simulink model "control"  (R2014a)
settings: Solver=ode1  StartTime=0.0  StopTime=inf  FixedStep=Ts  RelTol=1e-3
InitFcn:
  | control_initfcn
StopFcn:
  | control_stopfcn
values from neighbouring files (symbols this model uses):
  armSide = 0    [control_initfcn.m]
  dataLoggerStartTime = 1    [control_initfcn.m]
  dataLoggerStopTime = 100    [control_initfcn.m]
  forgettingFactor = 1e-2    (= 0.01)    [control_initfcn.m]
  g = [0 0 -9.81]'    [control_initfcn.m]
  initializationTime = timeForMovement + 4    (= 9)    [control_initfcn.m]
  initOrientationLeftArmTwo = [1 0 0 0]    [control_initfcn.m]
  initOrientationRightArmTwo = [1 0 0 0]    [control_initfcn.m]
  initPositionLeftArm = [0.7 0.23 1]    [control_initfcn.m]
  initPositionRightArm = [0.7 -0.23 1]    [control_initfcn.m]
  MANIPULATION_CMD_CONFIGURATION = 6    [control_initfcn.m]
  MANIPULATION_CMD_CONFIGURATION_VELOCITY = 102    [control_initfcn.m]
  maxTime = 10    [control_initfcn.m]
  minTime = 0.1    [control_initfcn.m]
  rampTime = 2    [control_initfcn.m]
  rotationAmplitude = [0.15;0;0.1462]    [control_initfcn.m]
  rotationFrequency = [0.5;0.6283;1.0472]    [control_initfcn.m]
  rotationPhaseShift = [pi;0;0]    [control_initfcn.m]
  timeForMovement = 5    [control_initfcn.m]
  translationAmplitude = 0*[0.005;0.02;0.01]    [control_initfcn.m]
  translationFrequency = [1.0472;0.6283;1.0472]    [control_initfcn.m]
  translationPhaseShift = [pi;0;0]    [control_initfcn.m]
  Ts = 0.01    [control_initfcn.m]
  vxMax = 0.5    [control_initfcn.m]
  vyMax = 0.5    [control_initfcn.m]
  vzMax = 0.5    [control_initfcn.m]
  wxMax = 0.5    [control_initfcn.m]
  wyMax = 0.5    [control_initfcn.m]
  wzMax = 0.5    [control_initfcn.m]
  xMax = 0.5 + offsetx    (= 1.2)    [control_initfcn.m]
  xMin = -0.1 + offsetx    (= 0.6)    [control_initfcn.m]
  yMax = 0.5 + offsety    (= 0.27)    [control_initfcn.m]
  yMin = -0.5 + offsety    (= -0.73)    [control_initfcn.m]
  zMax = 0.5 + offsetz    (= 1.4)    [control_initfcn.m]
  zMin = -0.5 + offsetz    (= 0.4)    [control_initfcn.m]
undefined symbols (not defined in the file or in its folder): cobot1a, qualisys, ws
libraries: dsparch4 x27, rtai_devices x22, sfbc_lib x6, simulink x2, rtai_utilities x2
settings Model: SimulationMode=external  Creator=wirnshofer  LastModifiedBy=bschmidt
settings DataIOCC: SignalLoggingSaveFormat=ModelDataLogs
settings RTWCC: SystemTargetFile=prt.tlc  TemplateMakefile=prt.tmf  Description=Linux PREEMPT_RT Real-Time Target  ProcessScript=prt_make_rtw_hook
settings STFCustomTargetCC: TargetLangStandard=C99 (ISO)  CodeReplacementLibrary=GNU C99 extensions  ModelReferenceCompliant=off  ConcurrentExecutionCompliant=off  MatFileLogging=on  SystemTargetFile=prt.tlc
settings GRTTargetCC: TargetLangStandard=C99 (ISO)  CodeReplacementLibrary=GNU C99 extensions  ModelReferenceCompliant=off  ParMdlRefBuildCompliant=off  CompOptLevelCompliant=off  ConcurrentExecutionCompliant=off  CombineOutputUpdateFcns=off  CPPClassGenCompliant=off  GRTInterface=on  ExtMode=on  ExtModeMexArgs='cobot1b'

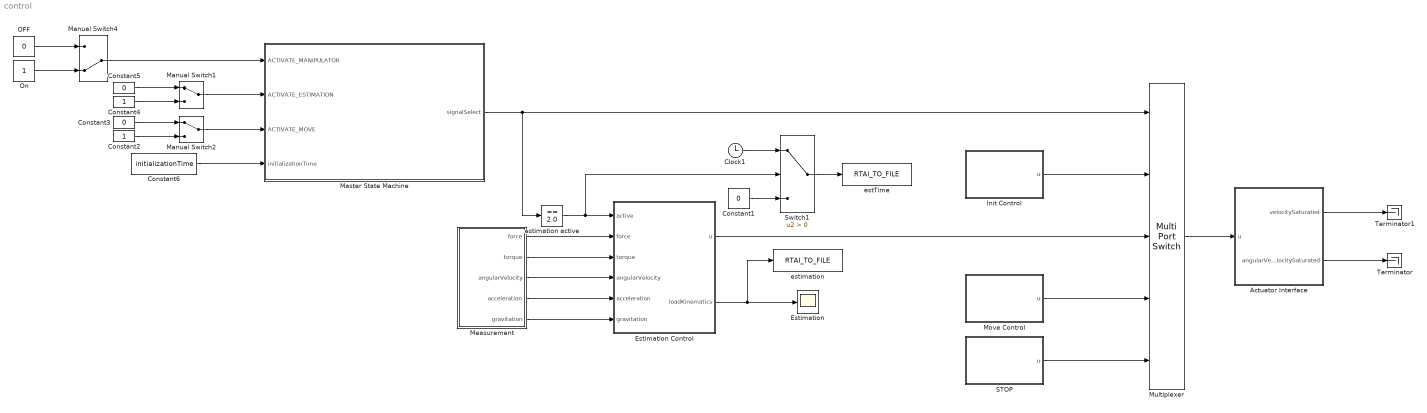
== system control ==
  Actuator Interface : Subsystem
  Clock1 : Clock
  Constant1 : Constant  Value=0
  Constant2 : Constant
  Constant3 : Constant  Value=0
  Constant4 : Constant
  Constant5 : Constant  Value=0
  Constant6 : Constant  Value=initializationTime
  Estimation : Scope
  Estimation Control : Subsystem
  Init Control : Subsystem
  Manual Switch1 : ManualSwitch
  Manual Switch2 : ManualSwitch
  Manual Switch4 : ManualSwitch  CurrentSetting=0
  Master State Machine : Stateflow chart  TreatAsAtomicUnit=on
  Measurement : Subsystem
  Move Control : Subsystem
  Multiplexer : MultiPortSwitch  Inputs=4
  OFF : Constant  Value=0
  On : Constant
  STOP : Subsystem
  Switch1 : Switch  Criteria=u2 > Threshold
  Terminator : Terminator
  Terminator1 : Terminator
  estTime : rtai_devices/RTAI_TO_FILE  N=1  InType=double  FileName='estTime.dat'  FpOutStr='%f '  TStartStop=[dataLoggerStartTime dataLoggerStopTime]  T=Ts  Confirm=off  Cutoff=off
  estimation : rtai_devices/RTAI_TO_FILE  N=10  InType=double  FileName='estimation.dat'  FpOutStr='%f '  TStartStop=[dataLoggerStartTime dataLoggerStopTime]  T=Ts  Confirm=off  Cutoff=off
  estimation active : simulink/Logic and Bit Operations/Compare To Constant  relop===  const=2.0  OutDataTypeStr=boolean
  wires:
  Init Control/1(u) -> Multiplexer/2
  Estimation Control/1(u) -> Multiplexer/3
  STOP/1(u) -> Multiplexer/5
  Move Control/1(u) -> Multiplexer/4
  Multiplexer/1 -> Actuator Interface/1(u)
  OFF/1 -> Manual Switch4/1
  On/1 -> Manual Switch4/2
  Manual Switch2/1 -> Master State Machine/3(ACTIVATE_MOVE)
  Constant3/1 -> Manual Switch2/1
  Constant2/1 -> Manual Switch2/2
  Estimation Control/2(loadKinematics) -> estimation/1, Estimation/1
  Measurement/1(force) -> Estimation Control/2(force)
  Measurement/2(torque) -> Estimation Control/3(torque)
  Measurement/5(gravitation) -> Estimation Control/6(gravitation)
  Measurement/3(angularVelocity) -> Estimation Control/4(angularVelocity)
  Actuator Interface/2(angularVelocitySaturated) -> Terminator/1
  Actuator Interface/1(velocitySaturated) -> Terminator1/1
  Measurement/4(acceleration) -> Estimation Control/5(acceleration)
  Manual Switch4/1 -> Master State Machine/1(ACTIVATE_MANIPULATOR)
  Switch1/1 -> estTime/1
  Manual Switch1/1 -> Master State Machine/2(ACTIVATE_ESTIMATION)
  Constant5/1 -> Manual Switch1/1
  Constant4/1 -> Manual Switch1/2
  Master State Machine/1(signalSelect) -> Multiplexer/1, estimation active/1
  estimation active/1 -> Switch1/2, Estimation Control/1(active)
  Constant1/1 -> Switch1/3
  Clock1/1 -> Switch1/1
  Constant6/1 -> Master State Machine/4(initializationTime)

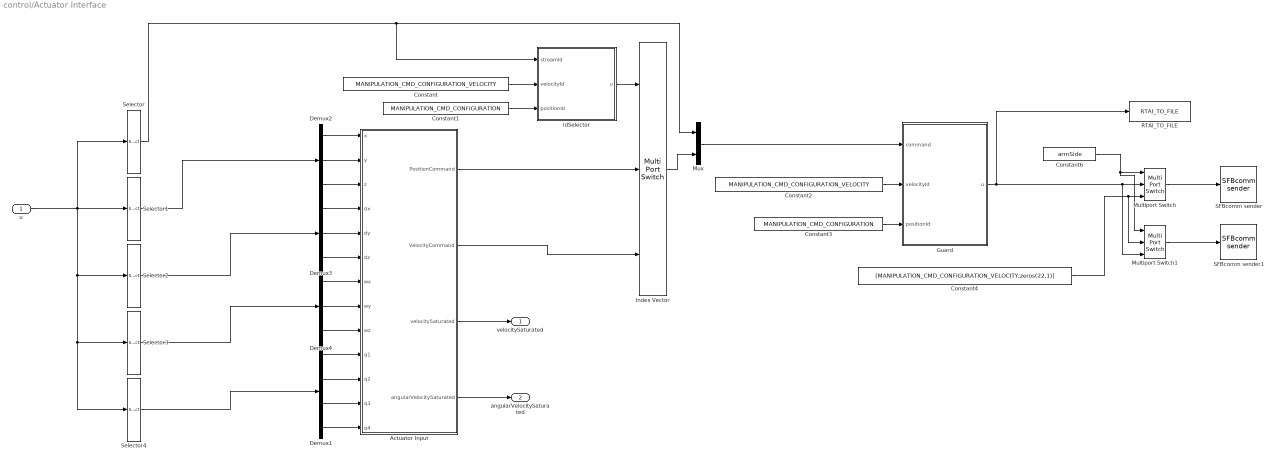
== system control/Actuator Interface ==
  u : Inport
  Actuator Input : Subsystem
  Constant : Constant  Value=MANIPULATION_CMD_CONFIGURATION_VELOCITY
  Constant1 : Constant  Value=MANIPULATION_CMD_CONFIGURATION
  Constant2 : Constant  Value=MANIPULATION_CMD_CONFIGURATION_VELOCITY
  Constant3 : Constant  Value=MANIPULATION_CMD_CONFIGURATION
  Constant4 : Constant  Value=[MANIPULATION_CMD_CONFIGURATION_VELOCITY;zeros(22,1)]
  Constant6 : Constant  Value=armSide
  Demux1 : Demux
  Demux2 : Demux  Outputs=3
  Demux3 : Demux  Outputs=3
  Demux4 : Demux  Outputs=3
  Guard : MATLAB Function  TreatAsAtomicUnit=on
  IdSelector : MATLAB Function  TreatAsAtomicUnit=on
  Index Vector : MultiPortSwitch  DataPortOrder=Zero-based contiguous  Inputs=2  zeroidx=on
  Multiport Switch : MultiPortSwitch  DataPortOrder=Zero-based contiguous  Inputs=2
  Multiport Switch1 : MultiPortSwitch  DataPortOrder=Zero-based contiguous  Inputs=2
  Mux : Mux  Inputs=2
  RTAI_TO_FILE : rtai_devices/RTAI_TO_FILE  N=23  InType=double  FileName='actContCmd.dat'  FpOutStr='%f '  TStartStop=[dataLoggerStartTime dataLoggerStopTime]  T=Ts  Confirm=off  Cutoff=off
  SFBcomm sender : sfbc_lib/SFBcomm sender  localPort=8566  streamID=2  remoteSettings=cobot1a:8565  portNames=A  connectTimeout=200  sampleTime=-1
  SFBcomm sender1 : sfbc_lib/SFBcomm sender  localPort=7566  streamID=2  remoteSettings=cobot1a:7565  portNames=A  connectTimeout=200  sampleTime=-1
  Selector : Selector  InputPortWidth=14
  Selector1 : Selector  InputPortWidth=14  Indices=[2:4]
  Selector2 : Selector  InputPortWidth=14  Indices=[5:7]
  Selector3 : Selector  InputPortWidth=14  Indices=[8:10]
  Selector4 : Selector  InputPortWidth=14  Indices=[11:14]
  velocitySaturated : Outport
  angularVelocitySaturated : Outport  Port=2
  wires:
  Constant/1 -> IdSelector/2(velocityId)
  Actuator Input/1(PositionCommand) -> Index Vector/2
  Constant1/1 -> IdSelector/3(positionId)
  Constant3/1 -> Guard/3(positionId)
  IdSelector/1(u) -> Index Vector/1
  Selector/1 -> IdSelector/1(streamId), Mux/1
  Mux/1 -> Guard/1(command)
  Index Vector/1 -> Mux/2
  Actuator Input/2(VelocityCommand) -> Index Vector/3
  Constant2/1 -> Guard/2(velocityId)
  u/1 -> Selector/1, Selector4/1, Selector3/1, Selector2/1, Selector1/1
  Demux2/3 -> Actuator Input/3(z)
  Demux2/1 -> Actuator Input/1(x)
  Demux2/2 -> Actuator Input/2(y)
  Demux3/1 -> Actuator Input/4(dx)
  Demux3/2 -> Actuator Input/5(dy)
  Demux3/3 -> Actuator Input/6(dz)
  Demux4/2 -> Actuator Input/8(wy)
  Demux4/1 -> Actuator Input/7(wx)
  Demux4/3 -> Actuator Input/9(wz)
  Selector1/1 -> Demux2/1
  Selector2/1 -> Demux3/1
  Selector3/1 -> Demux4/1
  Demux1/1 -> Actuator Input/10(q1)
  Demux1/2 -> Actuator Input/11(q2)
  Demux1/3 -> Actuator Input/12(q3)
  Demux1/4 -> Actuator Input/13(q4)
  Selector4/1 -> Demux1/1
  Actuator Input/3(velocitySaturated) -> velocitySaturated/1
  Actuator Input/4(angularVelocitySaturated) -> angularVelocitySaturated/1
  Multiport Switch1/1 -> SFBcomm sender1/1
  Guard/1(u) -> Multiport Switch1/3, Multiport Switch/2, RTAI_TO_FILE/1
  Multiport Switch/1 -> SFBcomm sender/1
  Constant4/1 -> Multiport Switch1/2, Multiport Switch/3
  Constant6/1 -> Multiport Switch1/1, Multiport Switch/1

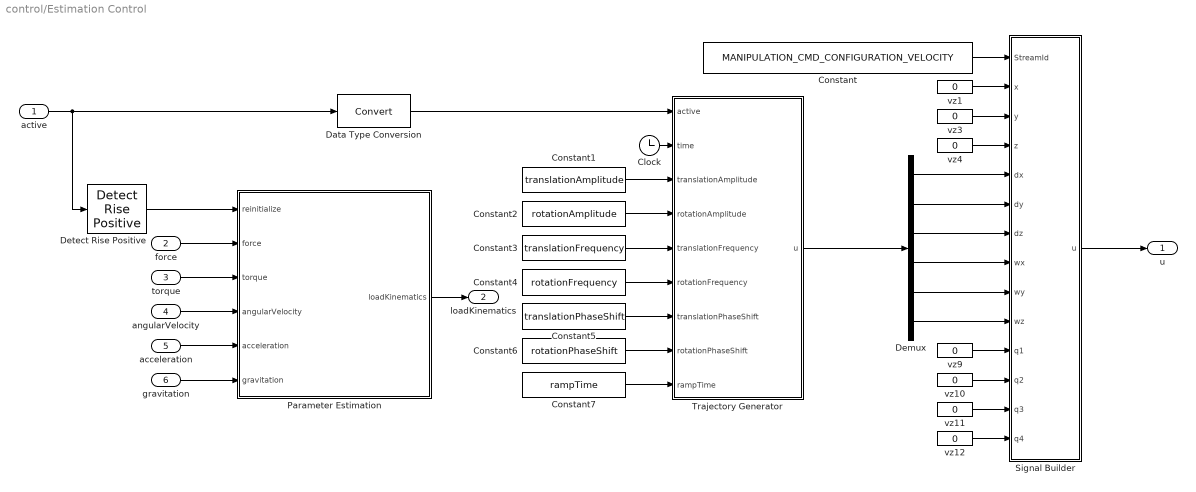
== system control/Estimation Control ==
  active : Inport
  force : Inport  Port=2
  torque : Inport  Port=3
  angularVelocity : Inport  Port=4
  acceleration : Inport  Port=5
  gravitation : Inport  Port=6
  Clock : Clock
  Constant : Constant  Value=MANIPULATION_CMD_CONFIGURATION_VELOCITY
  Constant1 : Constant  Value=translationAmplitude
  Constant2 : Constant  Value=rotationAmplitude
  Constant3 : Constant  Value=translationFrequency
  Constant4 : Constant  Value=rotationFrequency
  Constant5 : Constant  Value=translationPhaseShift
  Constant6 : Constant  Value=rotationPhaseShift
  Constant7 : Constant  Value=rampTime
  Data Type Conversion : DataTypeConversion
  Demux : Demux  Outputs=6
  Detect Rise Positive : simulink/Logic and Bit Operations/Detect Rise Positive  vinit=0  InputProcessing=Inherited  OutDataTypeStr=boolean
  Parameter Estimation : Subsystem
  Signal Builder : Subsystem
  Trajectory Generator : MATLAB Function  TreatAsAtomicUnit=on
  vz{1,3..4,9..12} (7 alike) : Constant  Value=0  SampleTime=Ts
  u : Outport
  loadKinematics : Outport  Port=2
  wires:
  active/1 -> Data Type Conversion/1, Detect Rise Positive/1
  Detect Rise Positive/1 -> Parameter Estimation/1(reinitialize)
  Constant/1 -> Signal Builder/1(StreamId)
  vz1/1 -> Signal Builder/2(x)
  vz3/1 -> Signal Builder/3(y)
  vz9/1 -> Signal Builder/11(q1)
  vz10/1 -> Signal Builder/12(q2)
  vz11/1 -> Signal Builder/13(q3)
  vz12/1 -> Signal Builder/14(q4)
  Signal Builder/1(u) -> u/1
  acceleration/1 -> Parameter Estimation/5(acceleration)
  angularVelocity/1 -> Parameter Estimation/4(angularVelocity)
  force/1 -> Parameter Estimation/2(force)
  torque/1 -> Parameter Estimation/3(torque)
  gravitation/1 -> Parameter Estimation/6(gravitation)
  Parameter Estimation/1(loadKinematics) -> loadKinematics/1
  vz4/1 -> Signal Builder/4(z)
  Clock/1 -> Trajectory Generator/2(time)
  Constant1/1 -> Trajectory Generator/3(translationAmplitude)
  Constant2/1 -> Trajectory Generator/4(rotationAmplitude)
  Constant6/1 -> Trajectory Generator/8(rotationPhaseShift)
  Constant3/1 -> Trajectory Generator/5(translationFrequency)
  Constant4/1 -> Trajectory Generator/6(rotationFrequency)
  Constant5/1 -> Trajectory Generator/7(translationPhaseShift)
  Constant7/1 -> Trajectory Generator/9(rampTime)
  Demux/6 -> Signal Builder/10(wz)
  Demux/5 -> Signal Builder/9(wy)
  Demux/4 -> Signal Builder/8(wx)
  Demux/3 -> Signal Builder/7(dz)
  Demux/2 -> Signal Builder/6(dy)
  Demux/1 -> Signal Builder/5(dx)
  Trajectory Generator/1(u) -> Demux/1
  Data Type Conversion/1 -> Trajectory Generator/1(active)

== system control/Init Control ==
  Constant : Constant  Value=armSide
  Constant1 : Constant  Value=initOrientationRightArmTwo
  Constant2 : Constant  Value=MANIPULATION_CMD_CONFIGURATION
  Constant3 : Constant  Value=zeros(6,1)
  Constant5 : Constant  Value=initPositionRightArm
  Constant6 : Constant  Value=initPositionLeftArm
  Constant7 : Constant  Value=initOrientationLeftArmTwo
  Demux : Demux  Outputs=3
  Demux1 : Demux  Outputs=6
  Demux2 : Demux
  Multiport Switch : MultiPortSwitch  DataPortOrder=Zero-based contiguous  Inputs=2
  Multiport Switch1 : MultiPortSwitch  DataPortOrder=Zero-based contiguous  Inputs=2
  Signal Builder : Subsystem
  u : Outport
  wires:
  Signal Builder/1(u) -> u/1
  Constant2/1 -> Signal Builder/1(StreamId)
  Demux/2 -> Signal Builder/3(y)
  Demux/1 -> Signal Builder/2(x)
  Demux/3 -> Signal Builder/4(z)
  Constant5/1 -> Multiport Switch/2
  Constant3/1 -> Demux1/1
  Constant1/1 -> Multiport Switch1/2
  Demux1/1 -> Signal Builder/5(dx)
  Demux1/2 -> Signal Builder/6(dy)
  Demux1/3 -> Signal Builder/7(dz)
  Demux1/4 -> Signal Builder/8(wx)
  Demux1/5 -> Signal Builder/9(wy)
  Demux1/6 -> Signal Builder/10(wz)
  Demux2/1 -> Signal Builder/11(q1)
  Demux2/2 -> Signal Builder/12(q2)
  Demux2/3 -> Signal Builder/13(q3)
  Demux2/4 -> Signal Builder/14(q4)
  Multiport Switch1/1 -> Demux2/1
  Multiport Switch/1 -> Demux/1
  Constant6/1 -> Multiport Switch/3
  Constant7/1 -> Multiport Switch1/3
  Constant/1 -> Multiport Switch1/1, Multiport Switch/1

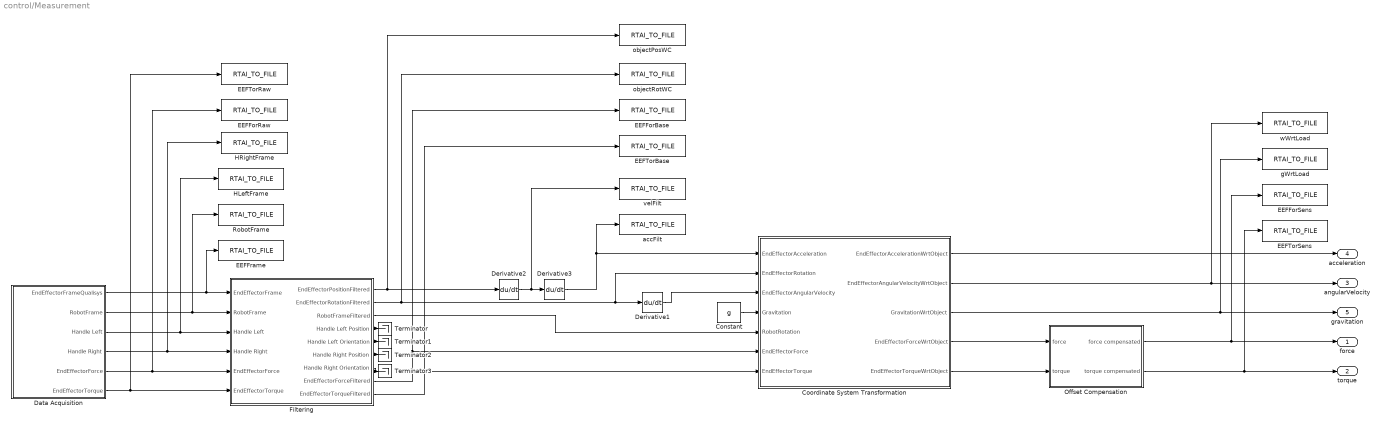
== system control/Measurement ==
  Constant : Constant  Value=g  SampleTime=-1
  Coordinate System Transformation : Subsystem
  Data Acquisition : Subsystem
  Derivative1 : Derivative
  Derivative2 : Derivative
  Derivative3 : Derivative
  EEFForBase : rtai_devices/RTAI_TO_FILE  N=3  InType=double  FileName='EEFForBase.dat'  FpOutStr='%f '  TStartStop=[dataLoggerStartTime dataLoggerStopTime]  T=Ts  Confirm=off  Cutoff=off
  EEFForRaw : rtai_devices/RTAI_TO_FILE  N=3  InType=double  FileName='EEFForRaw.dat'  FpOutStr='%f '  TStartStop=[dataLoggerStartTime dataLoggerStopTime]  T=Ts  Confirm=off  Cutoff=off
  EEFForSens : rtai_devices/RTAI_TO_FILE  N=3  InType=double  FileName='EEFForSens.dat'  FpOutStr='%f '  TStartStop=[dataLoggerStartTime dataLoggerStopTime]  T=Ts  Confirm=off  Cutoff=off
  EEFFrame : rtai_devices/RTAI_TO_FILE  N=8  InType=double  FileName='EEFFrame.dat'  FpOutStr='%f '  TStartStop=[dataLoggerStartTime dataLoggerStopTime]  T=Ts  Confirm=off  Cutoff=off
  EEFTorBase : rtai_devices/RTAI_TO_FILE  N=3  InType=double  FileName='EEFTorBase.dat'  FpOutStr='%f '  TStartStop=[dataLoggerStartTime dataLoggerStopTime]  T=Ts  Confirm=off  Cutoff=off
  EEFTorRaw : rtai_devices/RTAI_TO_FILE  N=3  InType=double  FileName='EEFTorRaw.dat'  FpOutStr='%f '  TStartStop=[dataLoggerStartTime dataLoggerStopTime]  T=Ts  Confirm=off  Cutoff=off
  EEFTorSens : rtai_devices/RTAI_TO_FILE  N=3  InType=double  FileName='EEFTorSens.dat'  FpOutStr='%f '  TStartStop=[dataLoggerStartTime dataLoggerStopTime]  T=Ts  Confirm=off  Cutoff=off
  Filtering : Subsystem
  HLeftFrame : rtai_devices/RTAI_TO_FILE  N=8  InType=double  FileName='HLeftFrame.dat'  FpOutStr='%f '  TStartStop=[dataLoggerStartTime dataLoggerStopTime]  T=Ts  Confirm=off  Cutoff=off
  HRightFrame : rtai_devices/RTAI_TO_FILE  N=8  InType=double  FileName='HRightFrame.dat'  FpOutStr='%f '  TStartStop=[dataLoggerStartTime dataLoggerStopTime]  T=Ts  Confirm=off  Cutoff=off
  Offset Compensation : Subsystem
  RobotFrame : rtai_devices/RTAI_TO_FILE  N=8  InType=double  FileName='RobotFrame.dat'  FpOutStr='%f '  TStartStop=[dataLoggerStartTime dataLoggerStopTime]  T=Ts  Confirm=off  Cutoff=off
  Terminator{,1..3} (4 alike) : Terminator
  accFilt : rtai_devices/RTAI_TO_FILE  N=3  InType=double  FileName='accFilt.dat'  FpOutStr='%f '  TStartStop=[dataLoggerStartTime dataLoggerStopTime]  T=Ts  Confirm=off  Cutoff=off
  gWrtLoad : rtai_devices/RTAI_TO_FILE  N=3  InType=double  FileName='gWrtLoad.dat'  FpOutStr='%f '  TStartStop=[dataLoggerStartTime dataLoggerStopTime]  T=Ts  Confirm=off  Cutoff=off
  objectPosWC : rtai_devices/RTAI_TO_FILE  N=3  InType=double  FileName='objectPosWC.dat'  FpOutStr='%f '  TStartStop=[dataLoggerStartTime dataLoggerStopTime]  T=Ts  Confirm=off  Cutoff=off
  objectRotWC : rtai_devices/RTAI_TO_FILE  N=3  InType=double  FileName='objectRotWC.dat'  FpOutStr='%f '  TStartStop=[dataLoggerStartTime dataLoggerStopTime]  T=Ts  Confirm=off  Cutoff=off
  velFilt : rtai_devices/RTAI_TO_FILE  N=3  InType=double  FileName='velFilt.dat'  FpOutStr='%f '  TStartStop=[dataLoggerStartTime dataLoggerStopTime]  T=Ts  Confirm=off  Cutoff=off
  wWrtLoad : rtai_devices/RTAI_TO_FILE  N=3  InType=double  FileName='wWrtLoad.dat'  FpOutStr='%f '  TStartStop=[dataLoggerStartTime dataLoggerStopTime]  T=Ts  Confirm=off  Cutoff=off
  force : Outport
  torque : Outport  Port=2
  angularVelocity : Outport  Port=3
  acceleration : Outport  Port=4
  gravitation : Outport  Port=5
  wires:
  Derivative2/1 -> Derivative3/1, velFilt/1
  Derivative3/1 -> Coordinate System Transformation/1(EndEffectorAcceleration), accFilt/1
  Filtering/9(EndEffectorTorqueFiltered) -> EEFTorBase/1, Coordinate System Transformation/7(EndEffectorTorque)
  Filtering/8(EndEffectorForceFiltered) -> EEFForBase/1, Coordinate System Transformation/6(EndEffectorForce)
  Filtering/1(EndEffectorPositionFiltered) -> Derivative2/1, objectPosWC/1
  Data Acquisition/1(EndEffectorFrameQualisys) -> EEFFrame/1, Filtering/1(EndEffectorFrame)
  Data Acquisition/2(RobotFrame) -> RobotFrame/1, Filtering/2(RobotFrame)
  Data Acquisition/5(EndEffectorForce) -> EEFForRaw/1, Filtering/5(EndEffectorForce)
  Data Acquisition/6(EndEffectorTorque) -> EEFTorRaw/1, Filtering/6(EndEffectorTorque)
  Coordinate System Transformation/2(EndEffectorAngularVelocityWrtObject) -> angularVelocity/1, wWrtLoad/1
  Coordinate System Transformation/3(GravitationWrtObject) -> gravitation/1, gWrtLoad/1
  Derivative1/1 -> Coordinate System Transformation/3(EndEffectorAngularVelocity)
  Constant/1 -> Coordinate System Transformation/4(Gravitation)
  Filtering/3(RobotFrameFiltered) -> Coordinate System Transformation/5(RobotRotation)
  Coordinate System Transformation/1(EndEffectorAccelerationWrtObject) -> acceleration/1
  Filtering/2(EndEffectorRotationFiltered) -> Derivative1/1, Coordinate System Transformation/2(EndEffectorRotation), objectRotWC/1
  Data Acquisition/3(Handle Left) -> HLeftFrame/1, Filtering/3(Handle Left)
  Data Acquisition/4(Handle Right) -> HRightFrame/1, Filtering/4(Handle Right)
  Filtering/4(Handle Left Position) -> Terminator/1
  Filtering/5(Handle Left Orientation) -> Terminator1/1
  Filtering/6(Handle Right Position) -> Terminator2/1
  Filtering/7(Handle Right Orientation) -> Terminator3/1
  Offset Compensation/2(torque compensated) -> EEFTorSens/1, torque/1
  Offset Compensation/1(force compensated) -> EEFForSens/1, force/1
  Coordinate System Transformation/4(EndEffectorForceWrtObject) -> Offset Compensation/1(force)
  Coordinate System Transformation/5(EndEffectorTorqueWrtObject) -> Offset Compensation/2(torque)

== system control/Move Control ==
  Constant : Constant  Value=MANIPULATION_CMD_CONFIGURATION_VELOCITY
  Signal Builder : Subsystem
  vz{,1..12} (13 alike) : Constant  Value=0  SampleTime=Ts
  u : Outport
  wires:
  vz/1 -> Signal Builder/2(x)
  vz2/1 -> Signal Builder/4(z)
  vz1/1 -> Signal Builder/3(y)
  Constant/1 -> Signal Builder/1(StreamId)
  Signal Builder/1(u) -> u/1
  vz3/1 -> Signal Builder/5(dx)
  vz8/1 -> Signal Builder/10(wz)
  vz5/1 -> Signal Builder/7(dz)
  vz4/1 -> Signal Builder/6(dy)
  vz7/1 -> Signal Builder/9(wy)
  vz6/1 -> Signal Builder/8(wx)
  vz12/1 -> Signal Builder/14(q4)
  vz9/1 -> Signal Builder/11(q1)
  vz11/1 -> Signal Builder/13(q3)
  vz10/1 -> Signal Builder/12(q2)

== system control/STOP ==
  Constant : Constant  Value=MANIPULATION_CMD_CONFIGURATION_VELOCITY
  Constant1 : Constant  Value=zeros(13,1)
  Demux : Demux  Outputs=13
  Signal Builder : Subsystem
  u : Outport
  wires:
  Signal Builder/1(u) -> u/1
  Constant/1 -> Signal Builder/1(StreamId)
  Demux/3 -> Signal Builder/4(z)
  Demux/6 -> Signal Builder/7(dz)
  Demux/1 -> Signal Builder/2(x)
  Demux/5 -> Signal Builder/6(dy)
  Demux/2 -> Signal Builder/3(y)
  Demux/7 -> Signal Builder/8(wx)
  Demux/9 -> Signal Builder/10(wz)
  Demux/8 -> Signal Builder/9(wy)
  Demux/4 -> Signal Builder/5(dx)
  Constant1/1 -> Demux/1
  Demux/10 -> Signal Builder/11(q1)
  Demux/11 -> Signal Builder/12(q2)
  Demux/12 -> Signal Builder/13(q3)
  Demux/13 -> Signal Builder/14(q4)

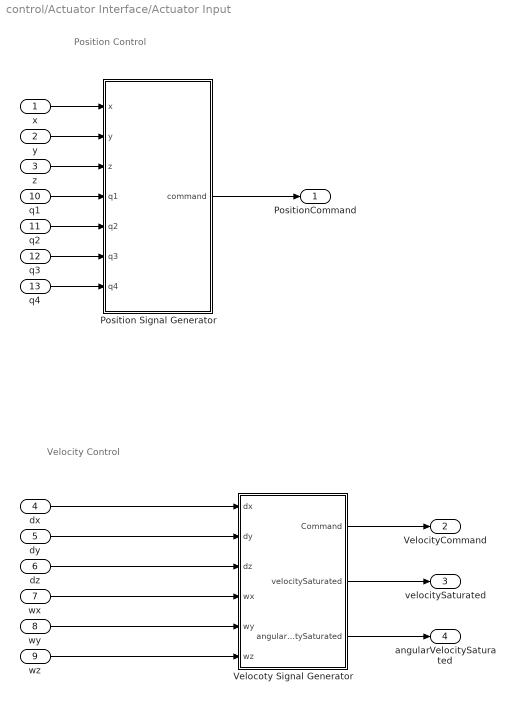
== system control/Actuator Interface/Actuator Input ==
  note: Velocity Control
  note: Position Control
  x : Inport
  y : Inport  Port=2
  z : Inport  Port=3
  dx : Inport  Port=4
  dy : Inport  Port=5
  dz : Inport  Port=6
  wx : Inport  Port=7
  wy : Inport  Port=8
  wz : Inport  Port=9
  q1 : Inport  Port=10
  q2 : Inport  Port=11
  q3 : Inport  Port=12
  q4 : Inport  Port=13
  Position Signal Generator : Subsystem
  Velocoty Signal Generator : Subsystem
  PositionCommand : Outport
  VelocityCommand : Outport  Port=2
  velocitySaturated : Outport  Port=3
  angularVelocitySaturated : Outport  Port=4
  wires:
  y/1 -> Position Signal Generator/2(y)
  Velocoty Signal Generator/1(Command) -> VelocityCommand/1
  wz/1 -> Velocoty Signal Generator/6(wz)
  z/1 -> Position Signal Generator/3(z)
  dx/1 -> Velocoty Signal Generator/1(dx)
  wx/1 -> Velocoty Signal Generator/4(wx)
  Position Signal Generator/1(command) -> PositionCommand/1
  wy/1 -> Velocoty Signal Generator/5(wy)
  dz/1 -> Velocoty Signal Generator/3(dz)
  dy/1 -> Velocoty Signal Generator/2(dy)
  x/1 -> Position Signal Generator/1(x)
  q1/1 -> Position Signal Generator/4(q1)
  q2/1 -> Position Signal Generator/5(q2)
  q3/1 -> Position Signal Generator/6(q3)
  q4/1 -> Position Signal Generator/7(q4)
  Velocoty Signal Generator/2(velocitySaturated) -> velocitySaturated/1
  Velocoty Signal Generator/3(angularVelocitySaturated) -> angularVelocitySaturated/1

== system control/Estimation Control/Parameter Estimation ==
  reinitialize : Inport
  force : Inport  Port=2
  torque : Inport  Port=3
  angularVelocity : Inport  Port=4
  acceleration : Inport  Port=5
  gravitation : Inport  Port=6
  Constant : Constant  Value=forgettingFactor
  Load Dynamics Estimation : MATLAB Function  TreatAsAtomicUnit=on
  anuglarAcceleration : Derivative
  loadKinematics : Outport
  wires:
  angularVelocity/1 -> Load Dynamics Estimation/3(omega), anuglarAcceleration/1
  acceleration/1 -> Load Dynamics Estimation/5(ddp)
  anuglarAcceleration/1 -> Load Dynamics Estimation/4(domega)
  Load Dynamics Estimation/1(thetaHat) -> loadKinematics/1
  force/1 -> Load Dynamics Estimation/1(F)
  torque/1 -> Load Dynamics Estimation/2(N)
  gravitation/1 -> Load Dynamics Estimation/6(g)
  Constant/1 -> Load Dynamics Estimation/7(forgettingFactor)
  reinitialize/1 -> Load Dynamics Estimation/8(reinitialize)

== system control/Estimation Control/Signal Builder ==
  StreamId : Inport
  x : Inport  Port=2
  y : Inport  Port=3
  z : Inport  Port=4
  dx : Inport  Port=5
  dy : Inport  Port=6
  dz : Inport  Port=7
  wx : Inport  Port=8
  wy : Inport  Port=9
  wz : Inport  Port=10
  q1 : Inport  Port=11
  q2 : Inport  Port=12
  q3 : Inport  Port=13
  q4 : Inport  Port=14
  Mux : Mux  Inputs=14
  u : Outport
  wires:
  Mux/1 -> u/1
  wy/1 -> Mux/9
  wx/1 -> Mux/8
  StreamId/1 -> Mux/1
  x/1 -> Mux/2
  dy/1 -> Mux/6
  dz/1 -> Mux/7
  dx/1 -> Mux/5
  z/1 -> Mux/4
  y/1 -> Mux/3
  wz/1 -> Mux/10
  q2/1 -> Mux/12
  q1/1 -> Mux/11
  q3/1 -> Mux/13
  q4/1 -> Mux/14

== system control/Init Control/Signal Builder ==
  StreamId : Inport
  x : Inport  Port=2
  y : Inport  Port=3
  z : Inport  Port=4
  dx : Inport  Port=5
  dy : Inport  Port=6
  dz : Inport  Port=7
  wx : Inport  Port=8
  wy : Inport  Port=9
  wz : Inport  Port=10
  q1 : Inport  Port=11
  q2 : Inport  Port=12
  q3 : Inport  Port=13
  q4 : Inport  Port=14
  Mux : Mux  Inputs=14
  u : Outport
  wires:
  Mux/1 -> u/1
  wy/1 -> Mux/9
  wx/1 -> Mux/8
  StreamId/1 -> Mux/1
  x/1 -> Mux/2
  dy/1 -> Mux/6
  dz/1 -> Mux/7
  dx/1 -> Mux/5
  z/1 -> Mux/4
  y/1 -> Mux/3
  wz/1 -> Mux/10
  q2/1 -> Mux/12
  q1/1 -> Mux/11
  q3/1 -> Mux/13
  q4/1 -> Mux/14

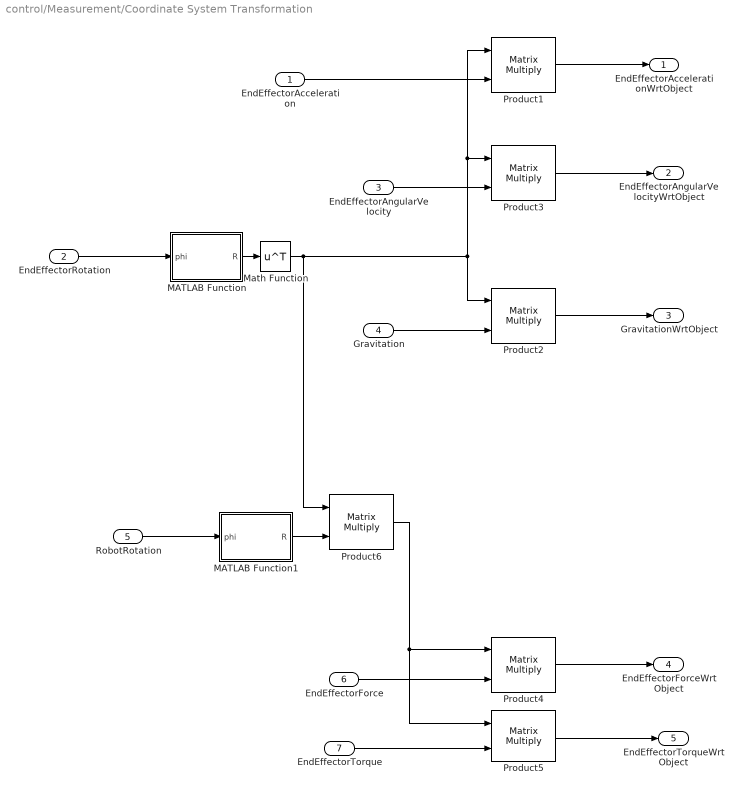
== system control/Measurement/Coordinate System Transformation ==
  EndEffectorAcceleration : Inport
  EndEffectorRotation : Inport  Port=2
  EndEffectorAngularVelocity : Inport  Port=3
  Gravitation : Inport  Port=4
  RobotRotation : Inport  Port=5
  EndEffectorForce : Inport  Port=6
  EndEffectorTorque : Inport  Port=7
  MATLAB Function : MATLAB Function  TreatAsAtomicUnit=on
  MATLAB Function1 : MATLAB Function  TreatAsAtomicUnit=on
  Math Function : Math  Operator=transpose  SaturateOnIntegerOverflow=on
  Product{1..6} (6 alike) : Product  Multiplication=Matrix(*)
  EndEffectorAccelerationWrtObject : Outport
  EndEffectorAngularVelocityWrtObject : Outport  Port=2
  GravitationWrtObject : Outport  Port=3
  EndEffectorForceWrtObject : Outport  Port=4
  EndEffectorTorqueWrtObject : Outport  Port=5
  wires:
  RobotRotation/1 -> MATLAB Function1/1(phi)
  EndEffectorTorque/1 -> Product5/2
  EndEffectorForce/1 -> Product4/2
  MATLAB Function/1(R) -> Math Function/1
  Product2/1 -> GravitationWrtObject/1
  Gravitation/1 -> Product2/2
  EndEffectorAngularVelocity/1 -> Product3/2
  Product3/1 -> EndEffectorAngularVelocityWrtObject/1
  Product1/1 -> EndEffectorAccelerationWrtObject/1
  Product4/1 -> EndEffectorForceWrtObject/1
  Product5/1 -> EndEffectorTorqueWrtObject/1
  Math Function/1 -> Product2/1, Product1/1, Product3/1, Product6/1
  MATLAB Function1/1(R) -> Product6/2
  Product6/1 -> Product5/1, Product4/1
  EndEffectorAcceleration/1 -> Product1/2
  EndEffectorRotation/1 -> MATLAB Function/1(phi)

== system control/Measurement/Data Acquisition ==
  Coordinate Rotation1 : Subsystem
  Coordinate Rotation2 : Subsystem
  Endeffector Measurement : Subsystem
  FH1 : rtai_utilities/RTAI debug  rate=1
  FH2 : rtai_utilities/RTAI debug  rate=1
  Human Grasp Measurement : Subsystem
  QualisysTracker : Subsystem
  EndEffectorFrameQualisys : Outport
  RobotFrame : Outport  Port=2
  Handle Left : Outport  Port=3
  Handle Right : Outport  Port=4
  EndEffectorForce : Outport  Port=5
  EndEffectorTorque : Outport  Port=6
  wires:
  Endeffector Measurement/1(EndeffectorForceWrtRobot) -> Coordinate Rotation1/1(Robot)
  Endeffector Measurement/2(EndeffectorTorqueWrtRobot) -> Coordinate Rotation2/1(Robot)
  Coordinate Rotation2/1(World) -> EndEffectorTorque/1
  Coordinate Rotation1/1(World) -> EndEffectorForce/1
  QualisysTracker/1(EndEffektorFrame) -> EndEffectorFrameQualisys/1
  QualisysTracker/2(RobotFrame) -> RobotFrame/1
  Human Grasp Measurement/1(Force H_1) -> FH1/1
  Human Grasp Measurement/3(Force H_2) -> FH2/1
  QualisysTracker/3(Handle Left) -> Handle Left/1
  QualisysTracker/4(Handle Right) -> Handle Right/1

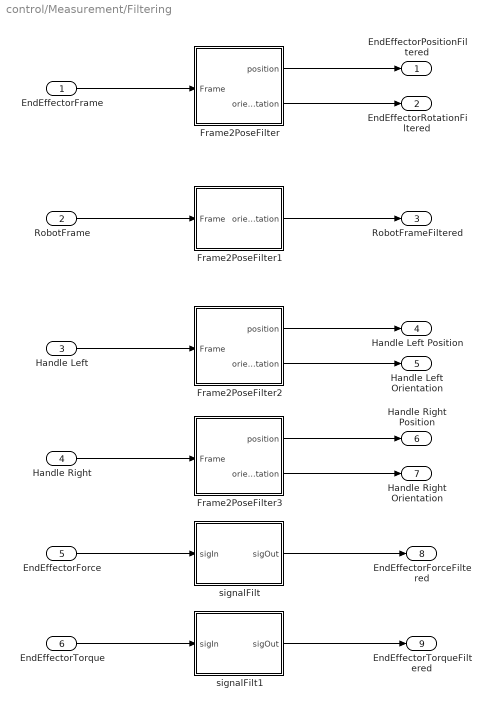
== system control/Measurement/Filtering ==
  EndEffectorFrame : Inport
  RobotFrame : Inport  Port=2
  Handle Left : Inport  Port=3
  Handle Right : Inport  Port=4
  EndEffectorForce : Inport  Port=5
  EndEffectorTorque : Inport  Port=6
  Frame2PoseFilter : Subsystem
  Frame2PoseFilter1 : Subsystem
  Frame2PoseFilter2 : Subsystem
  Frame2PoseFilter3 : Subsystem
  signalFilt : Subsystem
  signalFilt1 : Subsystem
  EndEffectorPositionFiltered : Outport
  EndEffectorRotationFiltered : Outport  Port=2
  RobotFrameFiltered : Outport  Port=3
  Handle Left Position : Outport  Port=4
  Handle Left Orientation : Outport  Port=5
  Handle Right Position : Outport  Port=6
  Handle Right Orientation : Outport  Port=7
  EndEffectorForceFiltered : Outport  Port=8
  EndEffectorTorqueFiltered : Outport  Port=9
  wires:
  RobotFrame/1 -> Frame2PoseFilter1/1(Frame)
  EndEffectorForce/1 -> signalFilt/1(sigIn)
  EndEffectorTorque/1 -> signalFilt1/1(sigIn)
  EndEffectorFrame/1 -> Frame2PoseFilter/1(Frame)
  Frame2PoseFilter/1(position) -> EndEffectorPositionFiltered/1
  Frame2PoseFilter1/1(orientation) -> RobotFrameFiltered/1
  signalFilt/1(sigOut) -> EndEffectorForceFiltered/1
  signalFilt1/1(sigOut) -> EndEffectorTorqueFiltered/1
  Frame2PoseFilter/2(orientation) -> EndEffectorRotationFiltered/1
  Handle Left/1 -> Frame2PoseFilter2/1(Frame)
  Frame2PoseFilter2/1(position) -> Handle Left Position/1
  Frame2PoseFilter2/2(orientation) -> Handle Left Orientation/1
  Handle Right/1 -> Frame2PoseFilter3/1(Frame)
  Frame2PoseFilter3/1(position) -> Handle Right Position/1
  Frame2PoseFilter3/2(orientation) -> Handle Right Orientation/1

== system control/Measurement/Offset Compensation ==
  force : Inport
  torque : Inport  Port=2
  Clock1 : Clock
  CompState : rtai_devices/RTAI_TO_FILE  N=1  InType=double  FileName='CompState.dat'  FpOutStr='%f '  TStartStop=[dataLoggerStartTime dataLoggerStopTime]  T=Ts  Confirm=off  Cutoff=off
  CompTrigg : rtai_devices/RTAI_TO_FILE  N=1  InType=double  FileName='CompTrigg.dat'  FpOutStr='%f '  TStartStop=[dataLoggerStartTime dataLoggerStopTime]  T=Ts  Confirm=off  Cutoff=off
  Constant1 : Constant  Value=timeForMovement + 2  SampleTime=-1
  Constant2 : Constant  Value=timeForMovement + 3  SampleTime=-1
  Data Type Conversion : DataTypeConversion
  Logical Operator : Logic  AllPortsSameDT=off  OutDataTypeStr=boolean
  MATLAB Function : MATLAB Function  TreatAsAtomicUnit=on
  Relational Operator : RelationalOperator  Operator=>  OutDataTypeStr=boolean
  Relational Operator1 : RelationalOperator  Operator=<  OutDataTypeStr=boolean
  force compensated : Outport
  torque compensated : Outport  Port=2
  wires:
  Relational Operator1/1 -> Logical Operator/2
  Constant1/1 -> Relational Operator/2
  MATLAB Function/2(Torque_Out) -> torque compensated/1
  Clock1/1 -> Relational Operator1/1, Relational Operator/1
  MATLAB Function/1(Force_Out) -> force compensated/1
  Relational Operator/1 -> Logical Operator/1
  Constant2/1 -> Relational Operator1/2
  force/1 -> MATLAB Function/2(Force)
  torque/1 -> MATLAB Function/3(Torque)
  Logical Operator/1 -> Data Type Conversion/1
  Data Type Conversion/1 -> CompTrigg/1, MATLAB Function/1(trigger)
  MATLAB Function/3(State) -> CompState/1

== system control/Move Control/Signal Builder ==
  StreamId : Inport
  x : Inport  Port=2
  y : Inport  Port=3
  z : Inport  Port=4
  dx : Inport  Port=5
  dy : Inport  Port=6
  dz : Inport  Port=7
  wx : Inport  Port=8
  wy : Inport  Port=9
  wz : Inport  Port=10
  q1 : Inport  Port=11
  q2 : Inport  Port=12
  q3 : Inport  Port=13
  q4 : Inport  Port=14
  Mux : Mux  Inputs=14
  u : Outport
  wires:
  Mux/1 -> u/1
  wy/1 -> Mux/9
  wx/1 -> Mux/8
  StreamId/1 -> Mux/1
  x/1 -> Mux/2
  dy/1 -> Mux/6
  dz/1 -> Mux/7
  dx/1 -> Mux/5
  z/1 -> Mux/4
  y/1 -> Mux/3
  wz/1 -> Mux/10
  q2/1 -> Mux/12
  q1/1 -> Mux/11
  q3/1 -> Mux/13
  q4/1 -> Mux/14

== system control/STOP/Signal Builder ==
  StreamId : Inport
  x : Inport  Port=2
  y : Inport  Port=3
  z : Inport  Port=4
  dx : Inport  Port=5
  dy : Inport  Port=6
  dz : Inport  Port=7
  wx : Inport  Port=8
  wy : Inport  Port=9
  wz : Inport  Port=10
  q1 : Inport  Port=11
  q2 : Inport  Port=12
  q3 : Inport  Port=13
  q4 : Inport  Port=14
  Mux : Mux  Inputs=14
  u : Outport
  wires:
  Mux/1 -> u/1
  wy/1 -> Mux/9
  wx/1 -> Mux/8
  StreamId/1 -> Mux/1
  x/1 -> Mux/2
  dy/1 -> Mux/6
  dz/1 -> Mux/7
  dx/1 -> Mux/5
  z/1 -> Mux/4
  y/1 -> Mux/3
  wz/1 -> Mux/10
  q2/1 -> Mux/12
  q1/1 -> Mux/11
  q3/1 -> Mux/13
  q4/1 -> Mux/14

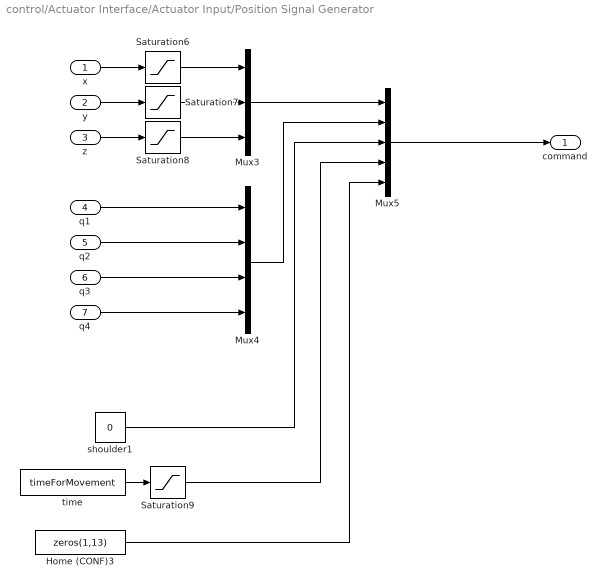
== system control/Actuator Interface/Actuator Input/Position Signal Generator ==
  x : Inport
  y : Inport  Port=2
  z : Inport  Port=3
  q1 : Inport  Port=4
  q2 : Inport  Port=5
  q3 : Inport  Port=6
  q4 : Inport  Port=7
  Home (CONF)3 : Constant  Value=zeros(1,13)  SampleTime=Ts
  Mux3 : Mux  Inputs=3
  Mux4 : Mux
  Mux5 : Mux  Inputs=5
  Saturation6 : Saturate  UpperLimit=xMax  LowerLimit=xMin
  Saturation7 : Saturate  UpperLimit=yMax  LowerLimit=yMin
  Saturation8 : Saturate  UpperLimit=zMax  LowerLimit=zMin
  Saturation9 : Saturate  UpperLimit=maxTime  LowerLimit=minTime
  shoulder1 : Constant  Value=0
  time : Constant  Value=timeForMovement
  command : Outport
  wires:
  z/1 -> Saturation8/1
  Mux3/1 -> Mux5/1
  Saturation7/1 -> Mux3/2
  Saturation9/1 -> Mux5/4
  Mux5/1 -> command/1
  Mux4/1 -> Mux5/2
  Saturation8/1 -> Mux3/3
  shoulder1/1 -> Mux5/3
  time/1 -> Saturation9/1
  Saturation6/1 -> Mux3/1
  x/1 -> Saturation6/1
  y/1 -> Saturation7/1
  Home (CONF)3/1 -> Mux5/5
  q1/1 -> Mux4/1
  q2/1 -> Mux4/2
  q3/1 -> Mux4/3
  q4/1 -> Mux4/4

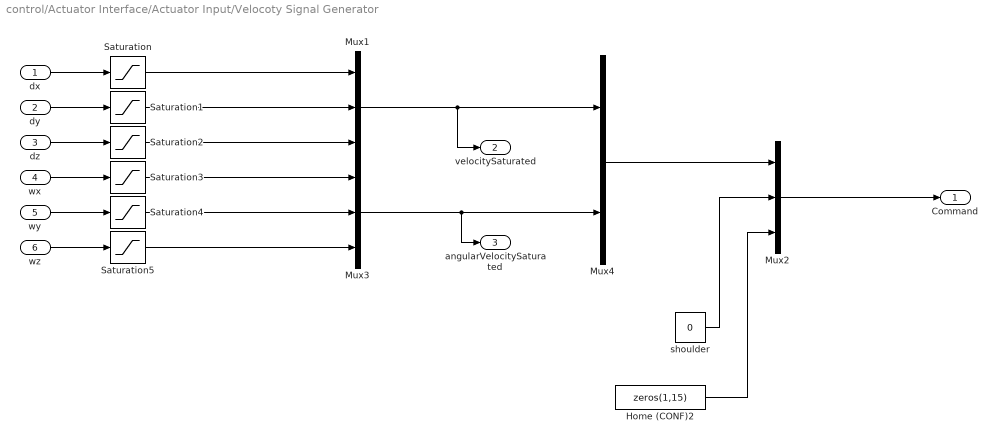
== system control/Actuator Interface/Actuator Input/Velocoty Signal Generator ==
  dx : Inport
  dy : Inport  Port=2
  dz : Inport  Port=3
  wx : Inport  Port=4
  wy : Inport  Port=5
  wz : Inport  Port=6
  Home (CONF)2 : Constant  Value=zeros(1,15)  SampleTime=Ts
  Mux1 : Mux  Inputs=3
  Mux2 : Mux  Inputs=3
  Mux3 : Mux  Inputs=3
  Mux4 : Mux  Inputs=2
  Saturation : Saturate  UpperLimit=vxMax  LowerLimit=-vxMax
  Saturation1 : Saturate  UpperLimit=vyMax  LowerLimit=-vyMax
  Saturation2 : Saturate  UpperLimit=vzMax  LowerLimit=-vzMax
  Saturation3 : Saturate  UpperLimit=wxMax  LowerLimit=-wxMax
  Saturation4 : Saturate  UpperLimit=wyMax  LowerLimit=-wyMax
  Saturation5 : Saturate  UpperLimit=wzMax  LowerLimit=-wzMax
  shoulder : Constant  Value=0
  Command : Outport
  velocitySaturated : Outport  Port=2
  angularVelocitySaturated : Outport  Port=3
  wires:
  wx/1 -> Saturation3/1
  Saturation3/1 -> Mux3/1
  dz/1 -> Saturation2/1
  Saturation/1 -> Mux1/1
  shoulder/1 -> Mux2/2
  wz/1 -> Saturation5/1
  wy/1 -> Saturation4/1
  dy/1 -> Saturation1/1
  Saturation2/1 -> Mux1/3
  Saturation1/1 -> Mux1/2
  Saturation5/1 -> Mux3/3
  Mux2/1 -> Command/1
  Saturation4/1 -> Mux3/2
  Mux4/1 -> Mux2/1
  dx/1 -> Saturation/1
  Home (CONF)2/1 -> Mux2/3
  Mux1/1 -> velocitySaturated/1, Mux4/1
  Mux3/1 -> angularVelocitySaturated/1, Mux4/2

== system control/Measurement/Data Acquisition/Coordinate Rotation1 ==
  Robot : Inport
  Demux3 : Demux  Outputs=3
  Gain2 : Gain  Gain=-1
  Mux : Mux  Inputs=3
  World : Outport
  wires:
  Mux/1 -> World/1
  Robot/1 -> Demux3/1
  Demux3/3 -> Mux/3
  Demux3/2 -> Gain2/1
  Demux3/1 -> Mux/2
  Gain2/1 -> Mux/1

== system control/Measurement/Data Acquisition/Coordinate Rotation2 ==
  Robot : Inport
  Demux3 : Demux  Outputs=3
  Gain2 : Gain  Gain=-1
  Mux : Mux  Inputs=3
  World : Outport
  wires:
  Mux/1 -> World/1
  Robot/1 -> Demux3/1
  Demux3/3 -> Mux/3
  Demux3/2 -> Gain2/1
  Demux3/1 -> Mux/2
  Gain2/1 -> Mux/1

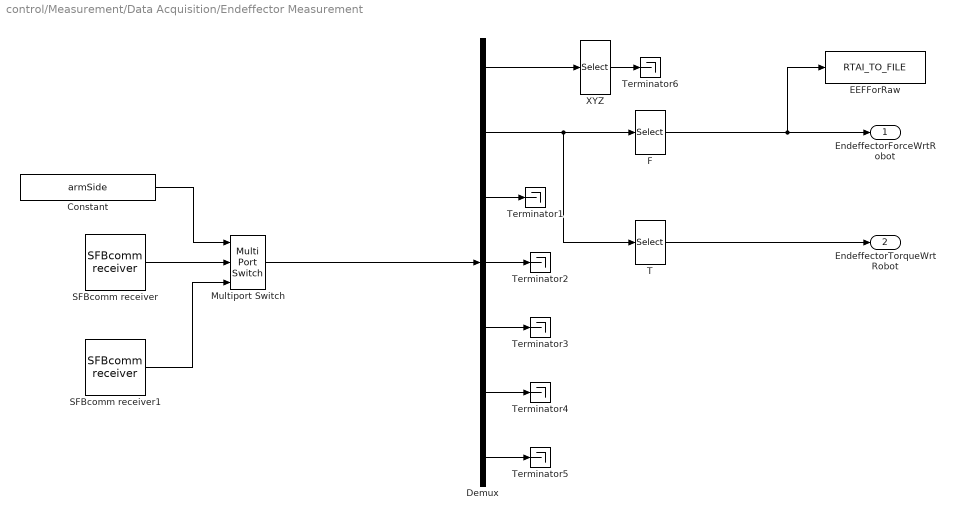
== system control/Measurement/Data Acquisition/Endeffector Measurement ==
  Constant : Constant  Value=armSide
  Demux : Demux  Outputs=[8 6 7 1 1 1 1]
  EEFForRaw : rtai_devices/RTAI_TO_FILE  N=3  InType=double  FileName='EEFForRaw.dat'  FpOutStr='%f '  TStartStop=[dataLoggerStartTime dataLoggerStopTime]  T=Ts  Confirm=off  Cutoff=off
  F : Selector  InputPortWidth=6  Indices=[1:3]
  Multiport Switch : MultiPortSwitch  DataPortOrder=Zero-based contiguous  Inputs=2
  SFBcomm receiver : sfbc_lib/SFBcomm receiver  localPort=8666  streamID=3  remoteSettings=cobot1a:8665  portNames=A  portWidths=25  outputLatency=off  outputIdleTime=off  connectTimeout=200  sampleTime=Ts
  SFBcomm receiver1 : sfbc_lib/SFBcomm receiver  localPort=7666  streamID=3  remoteSettings=cobot1a:7665  portNames=A  portWidths=25  outputLatency=off  outputIdleTime=off  connectTimeout=200  sampleTime=Ts
  T : Selector  InputPortWidth=6  Indices=[4:6]
  Terminator{1..6} (6 alike) : Terminator
  XYZ : Selector  InputPortWidth=8  Indices=[1:3]
  EndeffectorForceWrtRobot : Outport
  EndeffectorTorqueWrtRobot : Outport  Port=2
  wires:
  Demux/6 -> Terminator4/1
  Demux/7 -> Terminator5/1
  Demux/5 -> Terminator3/1
  Demux/4 -> Terminator2/1
  SFBcomm receiver/1 -> Multiport Switch/2
  Demux/1 -> XYZ/1
  Demux/3 -> Terminator1/1
  Demux/2 -> T/1, F/1
  F/1 -> EEFForRaw/1, EndeffectorForceWrtRobot/1
  T/1 -> EndeffectorTorqueWrtRobot/1
  SFBcomm receiver1/1 -> Multiport Switch/3
  Multiport Switch/1 -> Demux/1
  Constant/1 -> Multiport Switch/1
  XYZ/1 -> Terminator6/1

== system control/Measurement/Data Acquisition/Human Grasp Measurement ==
  Demux1 : Demux  Outputs=[ 3 3 3 3]
  SFBcomm receiver2 : sfbc_lib/SFBcomm receiver  localPort=14531  streamID=3  remoteSettings=qualisys-ws:1112  portNames=A  portWidths=12  outputLatency=off  outputIdleTime=off  connectTimeout=200  sampleTime=Ts
  Force H_1 : Outport
  Torque H_1 : Outport  Port=2
  Force H_2 : Outport  Port=3
  Torque H_2 : Outport  Port=4
  wires:
  SFBcomm receiver2/1 -> Demux1/1
  Demux1/1 -> Force H_1/1
  Demux1/2 -> Torque H_1/1
  Demux1/3 -> Force H_2/1
  Demux1/4 -> Torque H_2/1

== system control/Measurement/Data Acquisition/QualisysTracker ==
  SFBcomm receiver : sfbc_lib/SFBcomm receiver  localPort=33000  streamID=1  remoteSettings=127.0.0.1:34000  portNames=A  portWidths=32  outputLatency=off  outputIdleTime=off  connectTimeout=50  sampleTime=-1
  Selector : Selector  InputPortWidth=32  Indices=1:8
  Selector1 : Selector  InputPortWidth=32  Indices=9:16
  Selector2 : Selector  InputPortWidth=32  Indices=17:24
  Selector3 : Selector  InputPortWidth=32  Indices=25:32
  EndEffektorFrame : Outport
  RobotFrame : Outport  Port=2
  Handle Left : Outport  Port=3
  Handle Right : Outport  Port=4
  wires:
  SFBcomm receiver/1 -> Selector/1, Selector3/1, Selector2/1, Selector1/1
  Selector3/1 -> Handle Left/1
  Selector2/1 -> EndEffektorFrame/1
  Selector1/1 -> RobotFrame/1
  Selector/1 -> Handle Right/1

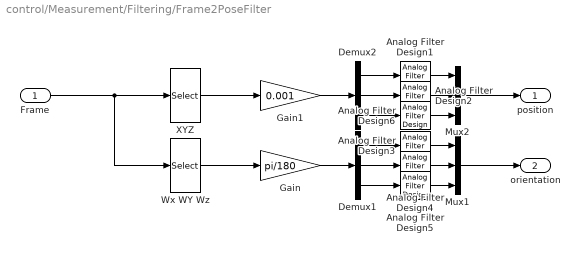
== system control/Measurement/Filtering/Frame2PoseFilter ==
  Frame : Inport
  Analog Filter Design{1..4} (4 alike) : dsparch4/Analog Filter Design  method=Butterworth  filttype=Lowpass  N=2  Wlo=cutOffFrequ  Whi=80  Rp=2  Rs=40
  Analog Filter Design5 : dsparch4/Analog Filter Design  method=Butterworth  filttype=Lowpass  N=3  Wlo=cutOffFrequ  Whi=80  Rp=2  Rs=40
  Analog Filter Design6 : dsparch4/Analog Filter Design  method=Butterworth  filttype=Lowpass  N=3  Wlo=cutOffFrequ  Whi=80  Rp=2  Rs=40
  Demux1 : Demux  Outputs=3
  Demux2 : Demux  Outputs=3
  Gain : Gain  Gain=pi/180
  Gain1 : Gain  Gain=0.001
  Mux1 : Mux  Inputs=3
  Mux2 : Mux  Inputs=3
  Wx WY Wz : Selector  InputPortWidth=8  Indices=[6:8]
  XYZ : Selector  InputPortWidth=8  Indices=[3:5]
  position : Outport
  orientation : Outport  Port=2
  wires:
  Wx WY Wz/1 -> Gain/1
  Frame/1 -> Wx WY Wz/1, XYZ/1
  XYZ/1 -> Gain1/1
  Demux1/1 -> Analog Filter Design3/1
  Demux1/2 -> Analog Filter Design4/1
  Demux1/3 -> Analog Filter Design5/1
  Analog Filter Design5/1 -> Mux1/3
  Analog Filter Design3/1 -> Mux1/1
  Analog Filter Design4/1 -> Mux1/2
  Demux2/1 -> Analog Filter Design1/1
  Demux2/2 -> Analog Filter Design2/1
  Demux2/3 -> Analog Filter Design6/1
  Gain/1 -> Demux1/1
  Mux1/1 -> orientation/1
  Gain1/1 -> Demux2/1
  Analog Filter Design6/1 -> Mux2/3
  Analog Filter Design1/1 -> Mux2/1
  Analog Filter Design2/1 -> Mux2/2
  Mux2/1 -> position/1

== system control/Measurement/Filtering/Frame2PoseFilter1 ==
  Frame : Inport
  Analog Filter Design3 : dsparch4/Analog Filter Design  method=Butterworth  filttype=Lowpass  N=2  Wlo=cutOffFrequ  Whi=80  Rp=2  Rs=40
  Analog Filter Design4 : dsparch4/Analog Filter Design  method=Butterworth  filttype=Lowpass  N=2  Wlo=cutOffFrequ  Whi=80  Rp=2  Rs=40
  Analog Filter Design5 : dsparch4/Analog Filter Design  method=Butterworth  filttype=Lowpass  N=3  Wlo=cutOffFrequ  Whi=80  Rp=2  Rs=40
  Demux1 : Demux  Outputs=3
  Gain : Gain  Gain=pi/180
  Mux1 : Mux  Inputs=3
  Wx WY Wz : Selector  InputPortWidth=8  Indices=[6:8]
  orientation : Outport
  wires:
  Wx WY Wz/1 -> Gain/1
  Frame/1 -> Wx WY Wz/1
  Demux1/1 -> Analog Filter Design3/1
  Demux1/2 -> Analog Filter Design4/1
  Demux1/3 -> Analog Filter Design5/1
  Analog Filter Design5/1 -> Mux1/3
  Analog Filter Design3/1 -> Mux1/1
  Analog Filter Design4/1 -> Mux1/2
  Gain/1 -> Demux1/1
  Mux1/1 -> orientation/1

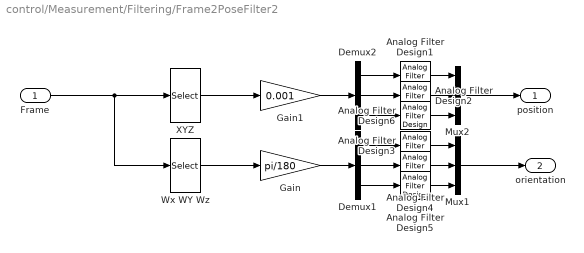
== system control/Measurement/Filtering/Frame2PoseFilter2 ==
  Frame : Inport
  Analog Filter Design{1..4} (4 alike) : dsparch4/Analog Filter Design  method=Butterworth  filttype=Lowpass  N=2  Wlo=cutOffFrequ  Whi=80  Rp=2  Rs=40
  Analog Filter Design5 : dsparch4/Analog Filter Design  method=Butterworth  filttype=Lowpass  N=3  Wlo=cutOffFrequ  Whi=80  Rp=2  Rs=40
  Analog Filter Design6 : dsparch4/Analog Filter Design  method=Butterworth  filttype=Lowpass  N=3  Wlo=cutOffFrequ  Whi=80  Rp=2  Rs=40
  Demux1 : Demux  Outputs=3
  Demux2 : Demux  Outputs=3
  Gain : Gain  Gain=pi/180
  Gain1 : Gain  Gain=0.001
  Mux1 : Mux  Inputs=3
  Mux2 : Mux  Inputs=3
  Wx WY Wz : Selector  InputPortWidth=8  Indices=[6:8]
  XYZ : Selector  InputPortWidth=8  Indices=[3:5]
  position : Outport
  orientation : Outport  Port=2
  wires:
  Wx WY Wz/1 -> Gain/1
  Frame/1 -> Wx WY Wz/1, XYZ/1
  XYZ/1 -> Gain1/1
  Demux1/1 -> Analog Filter Design3/1
  Demux1/2 -> Analog Filter Design4/1
  Demux1/3 -> Analog Filter Design5/1
  Analog Filter Design5/1 -> Mux1/3
  Analog Filter Design3/1 -> Mux1/1
  Analog Filter Design4/1 -> Mux1/2
  Demux2/1 -> Analog Filter Design1/1
  Demux2/2 -> Analog Filter Design2/1
  Demux2/3 -> Analog Filter Design6/1
  Gain/1 -> Demux1/1
  Mux1/1 -> orientation/1
  Gain1/1 -> Demux2/1
  Analog Filter Design6/1 -> Mux2/3
  Analog Filter Design1/1 -> Mux2/1
  Analog Filter Design2/1 -> Mux2/2
  Mux2/1 -> position/1

== system control/Measurement/Filtering/Frame2PoseFilter3 ==
  Frame : Inport
  Analog Filter Design{1..4} (4 alike) : dsparch4/Analog Filter Design  method=Butterworth  filttype=Lowpass  N=2  Wlo=cutOffFrequ  Whi=80  Rp=2  Rs=40
  Analog Filter Design5 : dsparch4/Analog Filter Design  method=Butterworth  filttype=Lowpass  N=3  Wlo=cutOffFrequ  Whi=80  Rp=2  Rs=40
  Analog Filter Design6 : dsparch4/Analog Filter Design  method=Butterworth  filttype=Lowpass  N=3  Wlo=cutOffFrequ  Whi=80  Rp=2  Rs=40
  Demux1 : Demux  Outputs=3
  Demux2 : Demux  Outputs=3
  Gain : Gain  Gain=pi/180
  Gain1 : Gain  Gain=0.001
  Mux1 : Mux  Inputs=3
  Mux2 : Mux  Inputs=3
  Wx WY Wz : Selector  InputPortWidth=8  Indices=[6:8]
  XYZ : Selector  InputPortWidth=8  Indices=[3:5]
  position : Outport
  orientation : Outport  Port=2
  wires:
  Wx WY Wz/1 -> Gain/1
  Frame/1 -> Wx WY Wz/1, XYZ/1
  XYZ/1 -> Gain1/1
  Demux1/1 -> Analog Filter Design3/1
  Demux1/2 -> Analog Filter Design4/1
  Demux1/3 -> Analog Filter Design5/1
  Analog Filter Design5/1 -> Mux1/3
  Analog Filter Design3/1 -> Mux1/1
  Analog Filter Design4/1 -> Mux1/2
  Demux2/1 -> Analog Filter Design1/1
  Demux2/2 -> Analog Filter Design2/1
  Demux2/3 -> Analog Filter Design6/1
  Gain/1 -> Demux1/1
  Mux1/1 -> orientation/1
  Gain1/1 -> Demux2/1
  Analog Filter Design6/1 -> Mux2/3
  Analog Filter Design1/1 -> Mux2/1
  Analog Filter Design2/1 -> Mux2/2
  Mux2/1 -> position/1

== system control/Measurement/Filtering/signalFilt ==
  sigIn : Inport
  Analog Filter Design1 : dsparch4/Analog Filter Design  method=Butterworth  filttype=Lowpass  N=2  Wlo=cutOffFrequ  Whi=80  Rp=2  Rs=40
  Analog Filter Design2 : dsparch4/Analog Filter Design  method=Butterworth  filttype=Lowpass  N=2  Wlo=cutOffFrequ  Whi=80  Rp=2  Rs=40
  Analog Filter Design6 : dsparch4/Analog Filter Design  method=Butterworth  filttype=Lowpass  N=3  Wlo=cutOffFrequ  Whi=80  Rp=2  Rs=40
  Demux2 : Demux  Outputs=3
  Mux2 : Mux  Inputs=3
  sigOut : Outport
  wires:
  Demux2/1 -> Analog Filter Design1/1
  Demux2/2 -> Analog Filter Design2/1
  Demux2/3 -> Analog Filter Design6/1
  Analog Filter Design6/1 -> Mux2/3
  Analog Filter Design1/1 -> Mux2/1
  Analog Filter Design2/1 -> Mux2/2
  Mux2/1 -> sigOut/1
  sigIn/1 -> Demux2/1

== system control/Measurement/Filtering/signalFilt1 ==
  sigIn : Inport
  Analog Filter Design1 : dsparch4/Analog Filter Design  method=Butterworth  filttype=Lowpass  N=2  Wlo=cutOffFrequ  Whi=80  Rp=2  Rs=40
  Analog Filter Design2 : dsparch4/Analog Filter Design  method=Butterworth  filttype=Lowpass  N=2  Wlo=cutOffFrequ  Whi=80  Rp=2  Rs=40
  Analog Filter Design6 : dsparch4/Analog Filter Design  method=Butterworth  filttype=Lowpass  N=3  Wlo=cutOffFrequ  Whi=80  Rp=2  Rs=40
  Demux2 : Demux  Outputs=3
  Mux2 : Mux  Inputs=3
  sigOut : Outport
  wires:
  Demux2/1 -> Analog Filter Design1/1
  Demux2/2 -> Analog Filter Design2/1
  Demux2/3 -> Analog Filter Design6/1
  Analog Filter Design6/1 -> Mux2/3
  Analog Filter Design1/1 -> Mux2/1
  Analog Filter Design2/1 -> Mux2/2
  Mux2/1 -> sigOut/1
  sigIn/1 -> Demux2/1

== stateflow chart control/Master State Machine ==
  state INIT_POSE_CONTROL
    during: signalSelect = 1;
  state ESTIMATION_CONTROL
    during: signalSelect = 2;
  state MOVE_CONTROL
    during: signalSelect = 3;
  state INIT
    during: signalSelect = 4;
  state STOP
    during: signalSelect = 4;
  INIT -> INIT_POSE_CONTROL : [ACTIVATE_MANIPULATOR == 1]
  INIT_POSE_CONTROL -> ESTIMATION_CONTROL [order 2] : [ACTIVATE_ESTIMATION == 1 && after(initializationTime,sec)]
  ESTIMATION_CONTROL -> MOVE_CONTROL [order 2] : [ACTIVATE_MOVE == 1]
  (default) -> INIT
  INIT_POSE_CONTROL -> STOP [order 1] : [ACTIVATE_MANIPULATOR == 0]
  ESTIMATION_CONTROL -> STOP [order 1] : [ACTIVATE_MANIPULATOR == 0 || ACTIVATE_ESTIMATION == 0]
  MOVE_CONTROL -> STOP : [ACTIVATE_MANIPULATOR == 0]
  data: ACTIVATE_MANIPULATOR input; signalSelect output; ACTIVATE_ESTIMATION input; ACTIVATE_MOVE input; initializationTime input

== matlab function control/Actuator Interface/Guard ==
  data: u output; command input; velocityId input; positionId input
function u = fcn(command,velocityId,positionId)



streamId = command(1);

if((streamId == velocityId || streamId == positionId) && length(command) == 23)
    u = command;
else
	u = [velocityId;zeros(22,1)];
end

== matlab function control/Estimation Control/Parameter Estimation/Load Dynamics Estimation ==
  data: F input; thetaHat output; N input; omega input; domega input; ddp input; g input; forgettingFactor input; reinitialize input
function thetaHat = fcn(F,N,omega,domega,ddp,g,forgettingFactor,reinitialize)
    thetaHat = estimationOneGraspingPoint(F,N,omega,domega,ddp,g,forgettingFactor,reinitialize);
end

== matlab function control/Measurement/Coordinate System Transformation/MATLAB Function ==
  data: phi input; R output
function R = fcn(phi)
    R = createRotationMatrix(phi);
end

== matlab function control/Actuator Interface/IdSelector ==
  data: streamId input; u output; velocityId input; positionId input
function u = fcn(streamId,velocityId,positionId)

switch(streamId)
    case velocityId
        u = 1;
    case positionId
        u = 0;
    otherwise
        u = 1;
end

== matlab function control/Measurement/Coordinate System Transformation/MATLAB Function1 ==
  data: phi input; R output
function R = fcn(phi)
    R = createRotationMatrix(phi);
end

== matlab function control/Measurement/Offset Compensation/MATLAB Function ==
  data: trigger input; Force_Out output; Force input; Torque input; Torque_Out output; State output
function [Force_Out, Torque_Out, State] = fcn(trigger,Force,Torque)
    persistent i previousTrigger currentState forceOffset torqueOffset;

    if isempty(i)
        i = 0;
    end
    if isempty(currentState)
        currentState = 0;
        % State 0 : output = input
        % State 1 : output = input && calculate 100 bin average
        % State 2 : output = input - offset
    end
    if isempty(previousTrigger)
        previousTrigger = 0;
    end
    if isempty(forceOffset)
        forceOffset = zeros(3, 1);
    end
    if isempty(torqueOffset)
        torqueOffset = zeros(3, 1);
    end
    
    
    %% Falling Edge
    if (previousTrigger==1 && trigger==0)
        currentState = 2;
    end
    %% Rising Edge
    if (previousTrigger==0 && trigger==1)
        currentState = 1;
        i = 0;
        forceOffset = 0;
        torqueOffset = 0;
    end
    
    if currentState == 1
        Force_Out = Force;
        Torque_Out = Torque;
        
        forceOffset = forceOffset + Force;
        torqueOffset = torqueOffset + Torque;
        i = i+1;
        
    elseif currentState == 2
        Force_Out = Force - forceOffset/i;
        Torque_Out = Torque - torqueOffset/i;
    else
        Force_Out = Force;
        Torque_Out = Torque;
    end
    previousTrigger = trigger;
    State = currentState;
end

== matlab function control/Estimation Control/Trajectory Generator ==
  data: active input; u output; time input; translationAmplitude input; rotationAmplitude input; translationFrequency input; rotationFrequency input; translationPhaseShift input; rotationPhaseShift input; rampTime input
function u  = fcn(active, time, translationAmplitude, rotationAmplitude, translationFrequency, rotationFrequency, translationPhaseShift, rotationPhaseShift, rampTime)

persistent timeOffset activePrevious;

if(isempty(timeOffset))
    timeOffset = 0;
end

if(isempty(activePrevious))
    activePrevious = 0;
end

if (active == 1 && activePrevious == 0)
    timeOffset = time;
end

if (active == 1)
    timeWithoutOffset = time - timeOffset;
    amplitudes = [translationAmplitude; rotationAmplitude];
    frequencies = [translationFrequency; rotationFrequency];
    phaseShifts = [translationPhaseShift; rotationPhaseShift];
    u = amplitudes.*sin(frequencies.*timeWithoutOffset + phaseShifts);
    
    if (timeWithoutOffset < rampTime)
        u = u*timeWithoutOffset/rampTime;
    end
else
    u = zeros(6, 1);
end

activePrevious = active;
